simulink model "BatteryEMA"  (R2022b)
settings: Solver=VariableStepAuto  StartTime=0.0  StopTime=10.0  RelTol=1e-3
undefined symbols (not defined in the file): param, SOCMPC, Subsystem
libraries: simulink x4
settings Model: Creator=davidworking  LastModifiedBy=davidworking

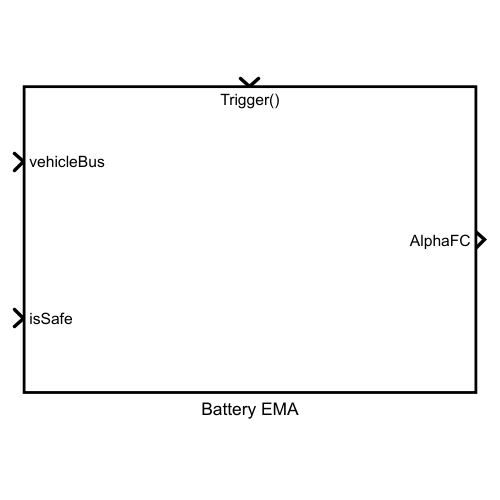
[thumbnail: Simulink's stored preview of the top-level diagram]
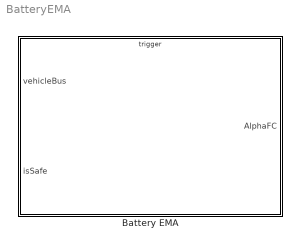
== system BatteryEMA ==
  Battery EMA : Subsystem

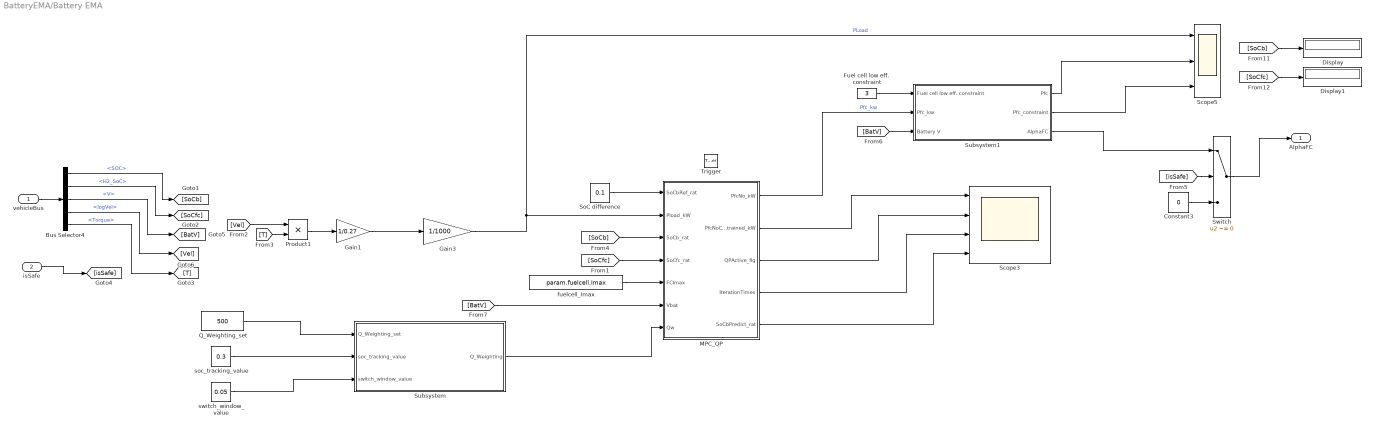
== system BatteryEMA/Battery EMA ==
  vehicleBus : Inport
  isSafe : Inport  Port=2
  Trigger : TriggerPort  TriggerType=function-call  VariantControl=(inherit)  PortDimensions=1
  Bus Selector4 : BusSelector  OutputSignals=batteryBus.SOC,rexBus.H2_SoC,batteryBus.V,chassisBus.logVel,chassisControlBus.Torque
  Constant3 : Constant  Value=0
  Display : Display
  Display1 : Display
  Fuel cell low eff. constraint : Constant  Value=3
  Gain1 : Gain  Gain=1/0.27
  Gain3 : Gain  Gain=1/1000
  MPC_QP : Subsystem  AncestorBlock=SOCMPC/Subsystem
      settings: LibrarySourceBlock=SOCMPC/Subsystem
  Product1 : Product
  Q_Weighting_set : Constant  Value=500
  Scope3 : Scope  NumInputPorts=4
  Scope5 : Scope  NumInputPorts=3
  SoC difference : Constant  Value=0.1
  Subsystem : Subsystem
  Subsystem1 : Subsystem
  Switch : Switch  Criteria=u2 ~= 0  SaturateOnIntegerOverflow=off  InputSameDT=off
  fuelcell_Imax : Constant  Value=param.fuelcell.Imax
  soc_tracking_value : Constant  Value=0.3
  switch_window_value : Constant  Value=0.05
  AlphaFC : Outport
  wires:
  Subsystem1/3(AlphaFC) -> Switch/1
  Subsystem1/1(Pfc) -> Scope5/2
  MPC_QP/1(PfcNo_kW) -> Subsystem1/2(Pfc_kw)  "Pfc_kw"
  [BatV] -> Subsystem1/3(Battery V)
  Subsystem/1(Q_Weighting) -> MPC_QP/7(Qw)
  Bus Selector4/5 -> [T]  "<Torque>"
  Bus Selector4/4 -> [Vel]  "<logVel>"
  [SoCb] -> MPC_QP/3(SoCb_rat)
  Fuel cell low eff. constraint/1 -> Subsystem1/1(Fuel cell low eff. constraint)
  [SoCfc] -> Display1/1
  Bus Selector4/3 -> [BatV]  "<V>"
  Bus Selector4/2 -> [SoCfc]  "<H2_SoC>"
  Gain1/1 -> Gain3/1
  Bus Selector4/1 -> [SoCb]  "<SOC>"
  [SoCfc] -> MPC_QP/4(SoCfc_rat)
  Constant3/1 -> Switch/3
  [BatV] -> MPC_QP/6(Vbat)
  MPC_QP/5(SoCbPredict_rat) -> Scope3/4
  fuelcell_Imax/1 -> MPC_QP/5(FCImax)
  MPC_QP/4(IterationTimes) -> Scope3/3
  [SoCb] -> Display/1
  [T] -> Product1/2
  SoC difference/1 -> MPC_QP/1(SoCbRef_rat)
  [Vel] -> Product1/1
  Switch/1 -> AlphaFC/1
  [isSafe] -> Switch/2
  MPC_QP/3(QPActive_flg) -> Scope3/2
  Gain3/1 -> MPC_QP/2(Pload_kW), Scope5/1  "PLoad"
  MPC_QP/2(PfcNoConstrained_kW) -> Scope3/1
  isSafe/1 -> [isSafe]
  soc_tracking_value/1 -> Subsystem/2(soc_tracking_value)
  vehicleBus/1 -> Bus Selector4/1
  switch_window_value/1 -> Subsystem/3(switch_window_value)
  Q_Weighting_set/1 -> Subsystem/1(Q_Weighting_set)
  Subsystem1/2(Pfc_constraint) -> Scope5/3
  Product1/1 -> Gain1/1

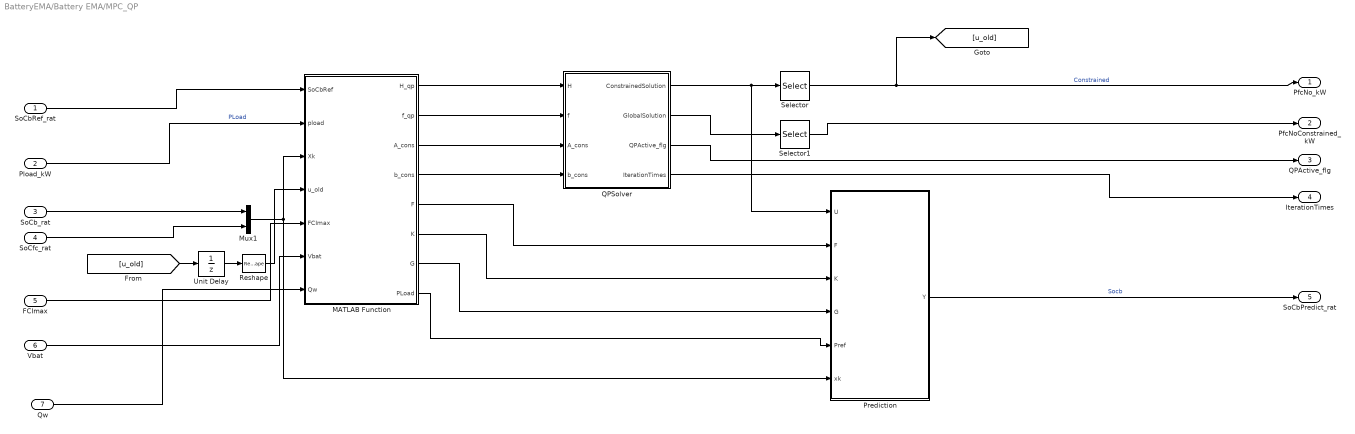
== system BatteryEMA/Battery EMA/MPC_QP ==
  SoCbRef_rat : Inport
  Pload_kW : Inport  Port=2
  SoCb_rat : Inport  Port=3
  SoCfc_rat : Inport  Port=4
  FCImax : Inport  Port=5
  Vbat : Inport  Port=6
  Qw : Inport  Port=7
  MATLAB Function : MATLAB Function  TreatAsAtomicUnit=on
  Mux1 : Mux  Inputs=2
  Prediction : MATLAB Function  TreatAsAtomicUnit=on
  QPSolver : Subsystem  mask{Size_H=3, N_u=3, iteration_max=30}
      mask prompts: Size_H "Hessian matrix size"; N_u "Number of target solution"; iteration_max "MaxIterations"
  Reshape : Reshape  OutputDimensionality=Column vector (2-D)
  Selector : Selector  IndexOptions=Index vector (dialog)  Indices=1  OutputSizes=1
  Selector1 : Selector  IndexOptions=Index vector (dialog)  Indices=1  OutputSizes=1
  Unit Delay : UnitDelay  SampleTime=-1  HasFrameUpgradeWarning=on
  PfcNo_kW : Outport
  PfcNoConstrained_kW : Outport  Port=2
  QPActive_flg : Outport  Port=3
  IterationTimes : Outport  Port=4
  SoCbPredict_rat : Outport  Port=5
  wires:
  Qw/1 -> MATLAB Function/7(Qw)
  Vbat/1 -> MATLAB Function/6(Vbat)
  FCImax/1 -> MATLAB Function/5(FCImax)
  Pload_kW/1 -> MATLAB Function/2(pload)  "PLoad"
  MATLAB Function/1(H_qp) -> QPSolver/1(H)
  Mux1/1 -> Prediction/6(xk), MATLAB Function/3(Xk)
  MATLAB Function/4(b_cons) -> QPSolver/4(b_cons)
  MATLAB Function/2(f_qp) -> QPSolver/2(f)
  Selector/1 -> [u_old], PfcNo_kW/1  "Constrained"
  MATLAB Function/7(G) -> Prediction/4(G)
  SoCb_rat/1 -> Mux1/1
  Reshape/1 -> MATLAB Function/4(u_old)
  MATLAB Function/3(A_cons) -> QPSolver/3(A_cons)
  QPSolver/1(ConstrainedSolution) -> Prediction/1(U), Selector/1
  MATLAB Function/6(K) -> Prediction/3(K)
  MATLAB Function/8(PLoad) -> Prediction/5(Pref)
  Unit Delay/1 -> Reshape/1
  QPSolver/2(GlobalSolution) -> Selector1/1
  Selector1/1 -> PfcNoConstrained_kW/1
  MATLAB Function/5(F) -> Prediction/2(F)
  [u_old] -> Unit Delay/1
  Prediction/1(Y) -> SoCbPredict_rat/1  "Socb"
  QPSolver/3(QPActive_flg) -> QPActive_flg/1
  QPSolver/4(IterationTimes) -> IterationTimes/1
  SoCbRef_rat/1 -> MATLAB Function/1(SoCbRef)
  SoCfc_rat/1 -> Mux1/2

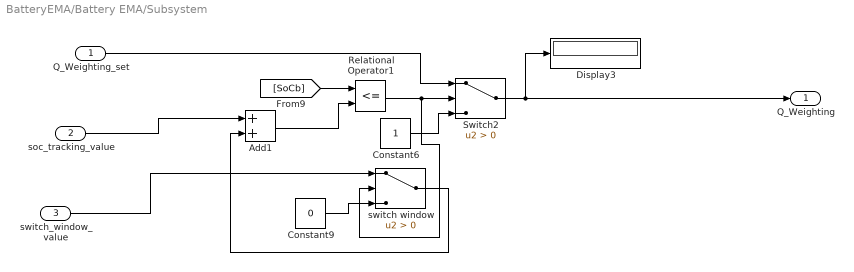
== system BatteryEMA/Battery EMA/Subsystem ==
  Q_Weighting_set : Inport
  soc_tracking_value : Inport  Port=2
  switch_window_value : Inport  Port=3
  Add1 : Sum
  Constant6 : Constant
  Constant9 : Constant  Value=0
  Display3 : Display
  Relational Operator1 : RelationalOperator  Operator=<=  OutDataTypeStr=boolean  RndMeth=Simplest  InputSameDT=off
  Switch2 : Switch  Criteria=u2 > Threshold  SaturateOnIntegerOverflow=off  InputSameDT=off
  switch window : Switch  Criteria=u2 > Threshold  SaturateOnIntegerOverflow=off  InputSameDT=off
  Q_Weighting : Outport
  wires:
  [SoCb] -> Relational Operator1/1
  Constant9/1 -> switch window/3
  Q_Weighting_set/1 -> Switch2/1
  Constant6/1 -> Switch2/3
  Relational Operator1/1 -> switch window/2, Switch2/2
  Switch2/1 -> Q_Weighting/1, Display3/1
  switch window/1 -> Add1/2
  Add1/1 -> Relational Operator1/2
  soc_tracking_value/1 -> Add1/1
  switch_window_value/1 -> switch window/1

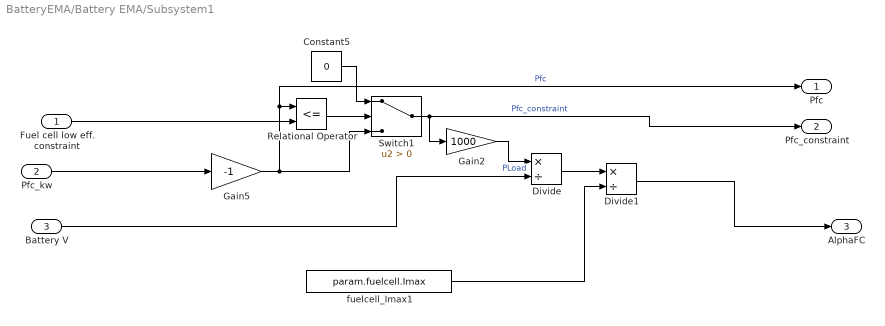
== system BatteryEMA/Battery EMA/Subsystem1 ==
  Fuel cell low eff. constraint : Inport
  Pfc_kw : Inport  Port=2
  Battery V : Inport  Port=3
  Constant5 : Constant  Value=0
  Divide : Product  Inputs=*/
  Divide1 : Product  Inputs=*/
  Gain2 : Gain  Gain=1000
  Gain5 : Gain  Gain=-1
  Relational Operator : RelationalOperator  Operator=<=  OutDataTypeStr=boolean  RndMeth=Simplest  InputSameDT=off
  Switch1 : Switch  Criteria=u2 > Threshold  SaturateOnIntegerOverflow=off  InputSameDT=off
  fuelcell_Imax1 : Constant  Value=param.fuelcell.Imax
  Pfc : Outport
  Pfc_constraint : Outport  Port=2
  AlphaFC : Outport  Port=3
  wires:
  Switch1/1 -> Pfc_constraint/1, Gain2/1  "Pfc_constraint"
  Divide1/1 -> AlphaFC/1
  Relational Operator/1 -> Switch1/2
  Pfc_kw/1 -> Gain5/1
  Divide/1 -> Divide1/1
  Constant5/1 -> Switch1/1
  fuelcell_Imax1/1 -> Divide1/2
  Gain5/1 -> Pfc/1, Relational Operator/1, Switch1/3  "Pfc"
  Gain2/1 -> Divide/1  "PLoad"
  Battery V/1 -> Divide/2
  Fuel cell low eff. constraint/1 -> Relational Operator/2

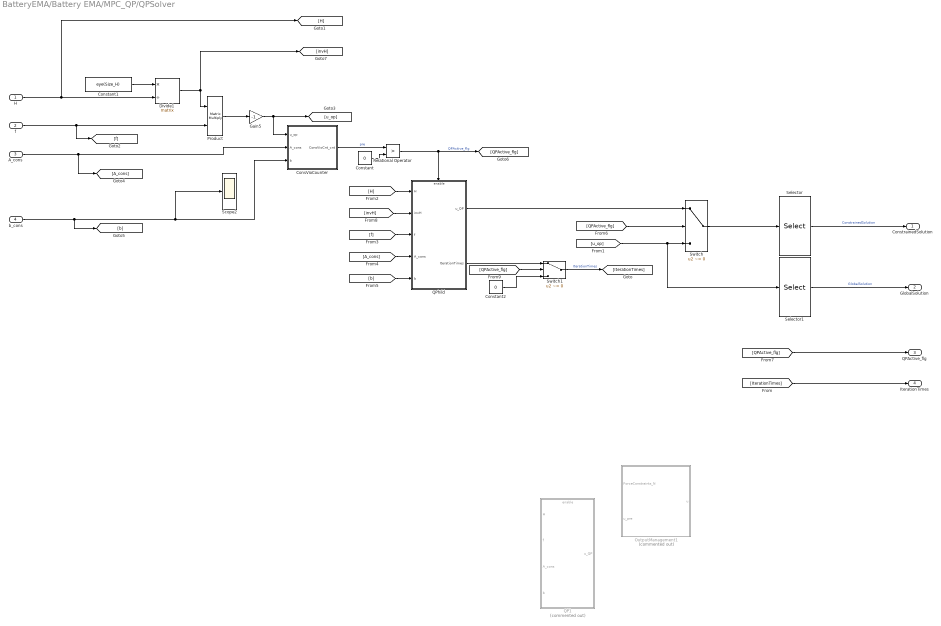
== system BatteryEMA/Battery EMA/MPC_QP/QPSolver ==
  H : Inport
  f : Inport  Port=2
  A_cons : Inport  Port=3
  b_cons : Inport  Port=4
  ConsVioCounter : Subsystem
  Constant : Constant  Value=0
  Constant1 : Constant  Value=eye(Size_H)
  Constant2 : Constant  Value=0
  Divide1 : Product  Inputs=*/  Multiplication=Matrix(*)
  Gain5 : Gain  Gain=-1
  OutputManagement1 : Subsystem  Commented=on
  Product : Product  Multiplication=Matrix(*)
  QP1 : Subsystem  Commented=on
  QPhild : Subsystem
  Relational Operator : RelationalOperator  Operator=>  OutDataTypeStr=boolean  RndMeth=Simplest  InputSameDT=off
  Scope2 : Scope
  Selector : Selector  IndexOptions=Index vector (dialog)  Indices=[1:N_u]  OutputSizes=1
  Selector1 : Selector  IndexOptions=Index vector (dialog)  Indices=[1:N_u]  OutputSizes=1
  Switch : Switch  Criteria=u2 ~= 0  SaturateOnIntegerOverflow=off  InputSameDT=off
  Switch1 : Switch  Criteria=u2 ~= 0  SaturateOnIntegerOverflow=off  InputSameDT=off
  ConstrainedSolution : Outport
  GlobalSolution : Outport  Port=2
  QPActive_flg : Outport  Port=3
  IterationTimes : Outport  Port=4
  wires:
  Selector1/1 -> GlobalSolution/1  "GlobalSolution"
  Selector/1 -> ConstrainedSolution/1  "ConstrainedSolution"
  f/1 -> Product/2, [f]
  A_cons/1 -> [A_cons], ConsVioCounter/2(A_cons)
  b_cons/1 -> [b], Scope2/1, ConsVioCounter/3(b)
  Product/1 -> Gain5/1
  Gain5/1 -> ConsVioCounter/1(u_op), [u_op]
  ConsVioCounter/1(ConsVioCnt_cnt) -> Relational Operator/1  "pre"
  Relational Operator/1 -> QPhild/Enable, [QPActive_flg]  "QPActive_flg"
  Constant/1 -> Relational Operator/2
  QPhild/1(u_QP) -> Switch/1
  [u_op] -> Selector1/1, Switch/3
  [H] -> QPhild/1(H)
  [f] -> QPhild/3(f)
  [A_cons] -> QPhild/4(A_cons)
  [b] -> QPhild/5(b)
  [QPActive_flg] -> Switch/2
  Switch/1 -> Selector/1
  [QPActive_flg] -> QPActive_flg/1
  Constant1/1 -> Divide1/1
  [invH] -> QPhild/2(invH)
  H/1 -> [H], Divide1/2
  Divide1/1 -> Product/1, [invH]
  [IterationTimes] -> IterationTimes/1
  Switch1/1 -> [IterationTimes]  "IterationTimes"
  QPhild/2(IterationTimes) -> Switch1/1
  [QPActive_flg] -> Switch1/2
  Constant2/1 -> Switch1/3

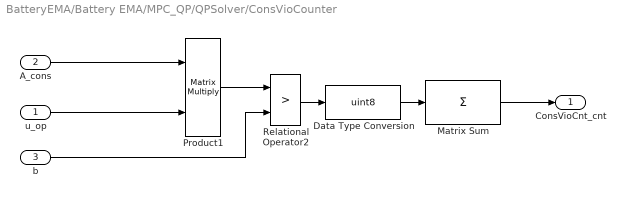
== system BatteryEMA/Battery EMA/MPC_QP/QPSolver/ConsVioCounter ==
  u_op : Inport
  A_cons : Inport  Port=2
  b : Inport  Port=3
  Data Type Conversion : DataTypeConversion  OutDataTypeStr=uint8  SaturateOnIntegerOverflow=off  RndMeth=Floor
  Matrix Sum : Sum  Inputs=+
  Product1 : Product  Multiplication=Matrix(*)
  Relational Operator2 : RelationalOperator  Operator=>  OutDataTypeStr=boolean  RndMeth=Simplest  InputSameDT=off
  ConsVioCnt_cnt : Outport
  wires:
  A_cons/1 -> Product1/1
  Relational Operator2/1 -> Data Type Conversion/1
  Data Type Conversion/1 -> Matrix Sum/1
  Product1/1 -> Relational Operator2/1
  u_op/1 -> Product1/2
  Matrix Sum/1 -> ConsVioCnt_cnt/1
  b/1 -> Relational Operator2/2

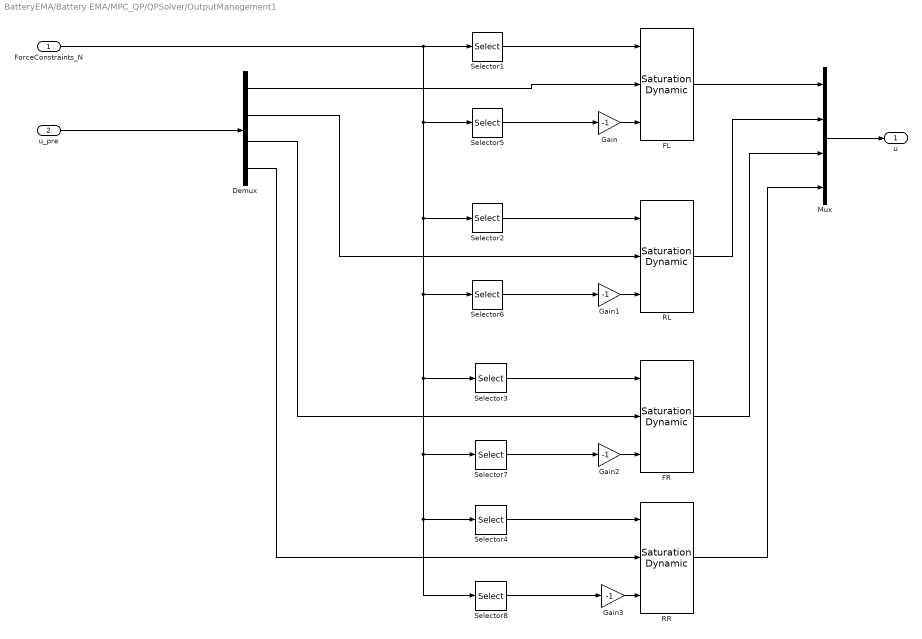
== system BatteryEMA/Battery EMA/MPC_QP/QPSolver/OutputManagement1 ==
  ForceConstraints_N : Inport
  u_pre : Inport  Port=2
  Demux : Demux
  FL : simulink/Discontinuities/Saturation Dynamic  OutMin=[]  OutMax=[]  OutDataTypeStr=Inherit: Same as second input  OutDataType=fixdt(1, 16)  OutScaling=2^-10  DoSatur=off
  FR : simulink/Discontinuities/Saturation Dynamic  OutMin=[]  OutMax=[]  OutDataTypeStr=Inherit: Same as second input  OutDataType=fixdt(1, 16)  OutScaling=2^-10  DoSatur=off
  Gain{,1..3} (4 alike) : Gain  Gain=-1
  Mux : Mux  Inputs=[1 1 1 1]
  RL : simulink/Discontinuities/Saturation Dynamic  OutMin=[]  OutMax=[]  OutDataTypeStr=Inherit: Same as second input  OutDataType=fixdt(1, 16)  OutScaling=2^-10  DoSatur=off
  RR : simulink/Discontinuities/Saturation Dynamic  OutMin=[]  OutMax=[]  OutDataTypeStr=Inherit: Same as second input  OutDataType=fixdt(1, 16)  OutScaling=2^-10  DoSatur=off
  Selector1 : Selector  InputPortWidth=8  IndexOptions=Index vector (dialog)  Indices=[5]  OutputSizes=1
  Selector2 : Selector  InputPortWidth=8  IndexOptions=Index vector (dialog)  Indices=6  OutputSizes=1
  Selector3 : Selector  InputPortWidth=8  IndexOptions=Index vector (dialog)  Indices=7  OutputSizes=1
  Selector4 : Selector  InputPortWidth=8  IndexOptions=Index vector (dialog)  Indices=8  OutputSizes=1
  Selector5 : Selector  InputPortWidth=8  IndexOptions=Index vector (dialog)  Indices=1  OutputSizes=1
  Selector6 : Selector  InputPortWidth=8  IndexOptions=Index vector (dialog)  Indices=2  OutputSizes=1
  Selector7 : Selector  InputPortWidth=8  IndexOptions=Index vector (dialog)  Indices=3  OutputSizes=1
  Selector8 : Selector  InputPortWidth=8  IndexOptions=Index vector (dialog)  Indices=4  OutputSizes=1
  u : Outport
  wires:
  Mux/1 -> u/1
  Selector5/1 -> Gain/1
  u_pre/1 -> Demux/1
  Selector7/1 -> Gain2/1
  Gain1/1 -> RL/3
  Demux/3 -> FR/2
  FL/1 -> Mux/1
  Selector4/1 -> RR/1
  Gain2/1 -> FR/3
  RL/1 -> Mux/2
  Selector8/1 -> Gain3/1
  Selector3/1 -> FR/1
  Gain3/1 -> RR/3
  Gain/1 -> FL/3
  Selector6/1 -> Gain1/1
  Demux/4 -> RR/2
  Demux/1 -> FL/2
  ForceConstraints_N/1 -> Selector4/1, Selector8/1, Selector7/1, Selector3/1, Selector6/1, Selector2/1, Selector5/1, Selector1/1
  Selector2/1 -> RL/1
  Selector1/1 -> FL/1
  Demux/2 -> RL/2
  FR/1 -> Mux/3
  RR/1 -> Mux/4

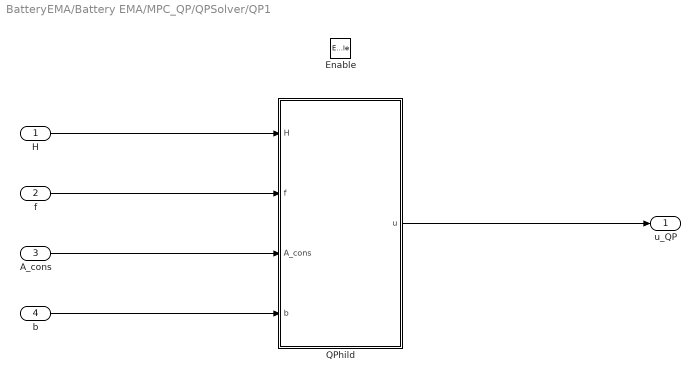
== system BatteryEMA/Battery EMA/MPC_QP/QPSolver/QP1 ==
  H : Inport
  f : Inport  Port=2
  A_cons : Inport  Port=3
  b : Inport  Port=4
  Enable : EnablePort
  QPhild : MATLAB Function  TreatAsAtomicUnit=on
  u_QP : Outport
  wires:
  QPhild/1(u) -> u_QP/1
  b/1 -> QPhild/4(b)
  A_cons/1 -> QPhild/3(A_cons)
  f/1 -> QPhild/2(f)
  H/1 -> QPhild/1(H)

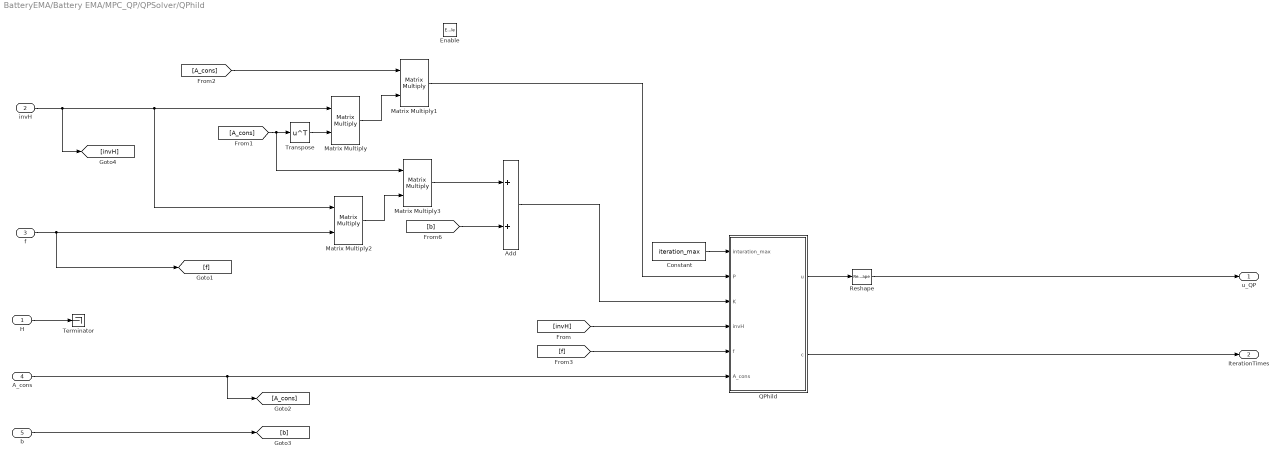
== system BatteryEMA/Battery EMA/MPC_QP/QPSolver/QPhild ==
  H : Inport  PortDimensions=[Size_H,Size_H]
  invH : Inport  Port=2  PortDimensions=[Size_H,Size_H]
  f : Inport  Port=3  PortDimensions=[Size_H,1]
  A_cons : Inport  Port=4
  b : Inport  Port=5
  Enable : EnablePort
  Add : Sum
  Constant : Constant  Value=iteration_max
  Matrix Multiply{,1..3} (4 alike) : Product  Multiplication=Matrix(*)
  QPhild : MATLAB Function  TreatAsAtomicUnit=on
  Reshape : Reshape  OutputDimensionality=Column vector (2-D)
  Terminator : Terminator
  Transpose : Math  Operator=transpose  SignedPower=on
  u_QP : Outport  PortDimensions=[Size_H,1]
  IterationTimes : Outport  Port=2  PortDimensions=[1,1]
  wires:
  QPhild/1(u) -> Reshape/1
  A_cons/1 -> [A_cons], QPhild/6(A_cons)
  b/1 -> [b]
  Matrix Multiply/1 -> Matrix Multiply1/2
  Transpose/1 -> Matrix Multiply/2
  [A_cons] -> Matrix Multiply1/1
  [A_cons] -> Matrix Multiply3/1, Transpose/1
  f/1 -> Matrix Multiply2/2, [f]
  Matrix Multiply2/1 -> Matrix Multiply3/2
  Matrix Multiply3/1 -> Add/1
  [b] -> Add/2
  Add/1 -> QPhild/3(K)
  Matrix Multiply1/1 -> QPhild/2(P)
  [f] -> QPhild/5(f)
  invH/1 -> [invH], Matrix Multiply2/1, Matrix Multiply/1
  H/1 -> Terminator/1
  [invH] -> QPhild/4(invH)
  QPhild/2(c) -> IterationTimes/1
  Constant/1 -> QPhild/1(interation_max)
  Reshape/1 -> u_QP/1

== matlab function BatteryEMA/Battery EMA/MPC_QP/MATLAB Function ==
  data: SoCbRef input; H_qp output; pload input; f_qp output; Xk input; u_old input; A_cons output; b_cons output; F output; K output; G output; PLoad output; FCImax input; Vbat input; Qw input
function [H_qp,f_qp,A_cons,b_cons,F,K,G,PLoad] = fcn(SoCbRef,pload,Xk,u_old,FCImax,Vbat,Qw)

%% Initialzization

% xk: SoC當下
% pload: demand power
% SoCbRef: 電池目標Soc


% vehicle parameters

C_b = 20; % 額定電池容量kwh
C_FC = 20; % 額定燃料電池容量kwh

% Prediction horizon /Control horizon/ Sample time
Np = 7;
Nc = 3;
Ts = 0.01;

% discretization
Ad = eye(2);
Bd = [-Ts/C_b/3600;
    Ts/C_FC/3600];
Dd=[Ts/(C_b*3600);0];
% output matrix
H= [1 -1];  
H1 = [0 1]; 

phi = Ad;
gamma = Bd;

B_CA = [-1 0 0;0 -1 0;0 0 -1];



% MPC initialization
NInp = 1;
NState = 2;

F = zeros(Np,NState);
F1 = zeros(Np,NState);
K = zeros(Np,Nc*NInp);
K1 = zeros(Np,Nc*NInp);
G = zeros(Np,Nc*1);


% Battery Soc
bufF = zeros(Np,NInp);
bufG = zeros(Np,1);
for j = 1:Np
    F(j,1:NState)=H*phi^j;
    bufF(j,1:NInp) = H*(phi^(j-1))*gamma;
    bufG(j,1:NInp) = H*(phi^(j-1))*Dd;
end

for i = 1:Nc
    K(i:Np,(1+(NInp)*(i-1):NInp*i)) = bufF(1:Np+1-i,:);
    G(i:Np,(1+(NInp)*(i-1):NInp*i)) = bufG(1:Np+1-i,:);
end


% Fuel cell Soc
% Load power has nothing to do with fuel cell SoC. Therefore, the
% distrubance matrix G1 is neglected in fuel cell prediction

bufF = zeros(Np,NInp);
for j = 1:Np
    F1(j,1:NState)=H1*phi^j;
    bufF(j,1:NInp) = H1*(phi^(j-1))*gamma;
end

for i = 1:Nc
    K1(i:Np,(1+(NInp)*(i-1):NInp*i)) = bufF(1:Np+1-i,:);
end




%% MPC constraints

% amplitude constraint on control signal
umin = -(FCImax*Vbat)/1000;  % Fuel cell discharge
umax = 0; % Fuel cell cannot be charged
Umin = repmat(umin,Nc,1);
Umax = repmat(umax,Nc,1);


M2=[-eye(Nc*NInp); eye(Nc*NInp)];
N2 = [-Umin; Umax];

A_cons = M2;
b_cons = N2;


%% Weighting

% change rate weighting
Adeltau = eye(Nc*NInp,Nc*NInp);

for i=1:Nc*NInp-NInp
    Adeltau(i+NInp,i) = -1;
end
Aold = [-1*eye(NInp,NInp);zeros((Nc-1)*NInp,NInp)];



% use Brison's rule to determine the first pair of weightings
SoC_max_err = 0.03; % maximum allowable SoC tracking error
Pmax =  10; % kW, maximum allowable power
Pdelta_max =  0.2; % kW, maximum allowable power change rate

Q = Qw*eye(Np)/SoC_max_err^2;  % SoC tracking weighting
R_bar = 0.1*eye(Nc)/Pmax^2;   % Control input weighting
R_delta = 0*eye(Nc)/Pdelta_max^2;   % Change rate weighting

rho = 1; % Pload tracking weighting

Yref = SoCbRef*ones(Np,1);
PLoad = pload*ones(Nc,1);


%% old
% H_qp =  (K')*Q*K  + R_bar  + rho*(B_CA')*B_CA +(Adeltau')*R_delta*Adeltau;
% H_qp = (H_qp+H_qp')/2;
% f_qp = -( (K')*Q*(Yref-F*Xk)   + rho*(B_CA')*PLoad + (Adeltau')*R_delta*Aold*u_old );


%% new
H_qp =  (K')*Q*K  + R_bar  + rho*(B_CA')*B_CA +(Adeltau')*R_delta*Adeltau;
H_qp = (H_qp+H_qp')/2;
f_qp = -( (K')*Q*(Yref-F*Xk) + (K')*Q*G*PLoad  + rho*(B_CA')*PLoad + (Adeltau')*R_delta*Aold*u_old );

== matlab function BatteryEMA/Battery EMA/MPC_QP/QPSolver/QP1/QPhild ==
  data: u output; H input; f input; A_cons input; b input
function u  = QPhild(H,f,A_cons,b)

%% Procedure start
P=A_cons*(H\A_cons');
K=(A_cons*(H\f)+b);

[n,m]=size(K);  % n is the number of the constraints.
x_ini=zeros(n,m);
lambda=x_ini;
al=10;
interation_max = 10;

for km=1:interation_max
%     find the elements in the solution vector one by one
%     km could be larger if the Lagranger multiplier has a slow
%     convergence rate.
    
    lambda_p=lambda;
    
    for i=1:n
        w= P(i,:)*lambda-P(i,i)*lambda(i,1);
        w=w+K(i,1);
        la=-w/P(i,i);
        lambda(i,1)=max(0,la);
    end
    al=(lambda-lambda_p)'*(lambda-lambda_p);

    if (al<10e-8); break; end

end

u = -H\(f + A_cons'*lambda);

end

== matlab function BatteryEMA/Battery EMA/MPC_QP/QPSolver/QPhild/QPhild ==
  data: interation_max input; P input; K input; u output; invH input; f input; A_cons input; c output
    function [u,c]  = QPhild(interation_max,P,K,invH,f,A_cons)
%% Procedure start
[n,m]=size(K);  % n is the number of the constraints.
x_ini=zeros(n,m);
lambda=x_ini;
al=10;
c=0;
for km=1:interation_max
    c=c+1;
%     find the elements in the solution vector one by one
%     km could be larger if the Lagranger multiplier has a slow
%     convergence rate.
    
    lambda_p=lambda;
    
    for i=1:n
        w= P(i,:)*lambda-P(i,i)*lambda(i,1);
        w=w+K(i,1);
        la=-w/P(i,i);
        lambda(i,1)=max(0,la);
    end
    al=(lambda-lambda_p)'*(lambda-lambda_p);

    if (al<10e-8); break; end

end

u = -invH*(f + A_cons'*lambda);

end

== matlab function BatteryEMA/Battery EMA/MPC_QP/Prediction ==
  data: U input; Y output; F input; K input; G input; Pref input; xk input
function Y = fcn(U,F,K,G,Pref,xk)



Y=F*xk+K*U+G*Pref;
